simulink model "lab3s"  (R2025a)
settings: Solver=VariableStepAuto  StartTime=0.0  StopTime=15  MaxStep=5e-4  RelTol=1e-3
InitFcn:
  | clear;
  | 
  | % Plant Parameters
  | A = [0 1;-15 -7];
  | b0 = 3;
  | b = [0;3];
  | 
  | % Reference Model Parameters
  | c= 2;
  | tTa = 4.74;
  | tT= 0.7;
  | omega0 = tTa/tT;
  | 
  | am0 = omega0^2;
  | am1 = c * omega0;
  | Am = [0 1;-am0 -am1];
  | bm0 = am0;
  | bm = [0;bm0];
  | 
  | C = eye(2);
  | Q = eye(2);
  | 
  | % Controller Parameters
  | gamma =1;
  | P = lyap(Am',Q);
  | 
  | 
  | theta1 = (-am1 + A(2,1))/b0;
  | theta2 = (-am0 + A(2,2))/b0;
  | theta = [theta1;theta2];
settings Model: SimulationMode=accelerator  Creator=zuimio  LastModifiedBy=zuimio

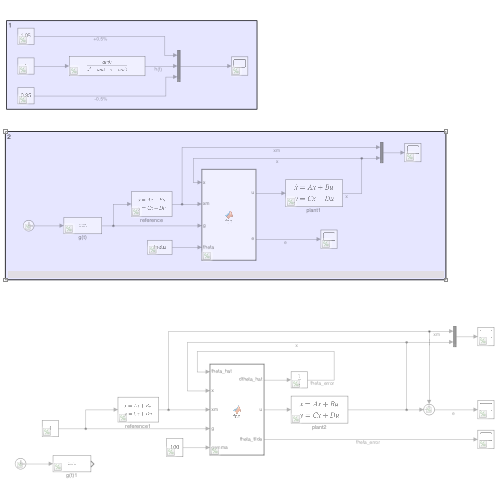
[thumbnail: Simulink's stored preview of the top-level diagram]
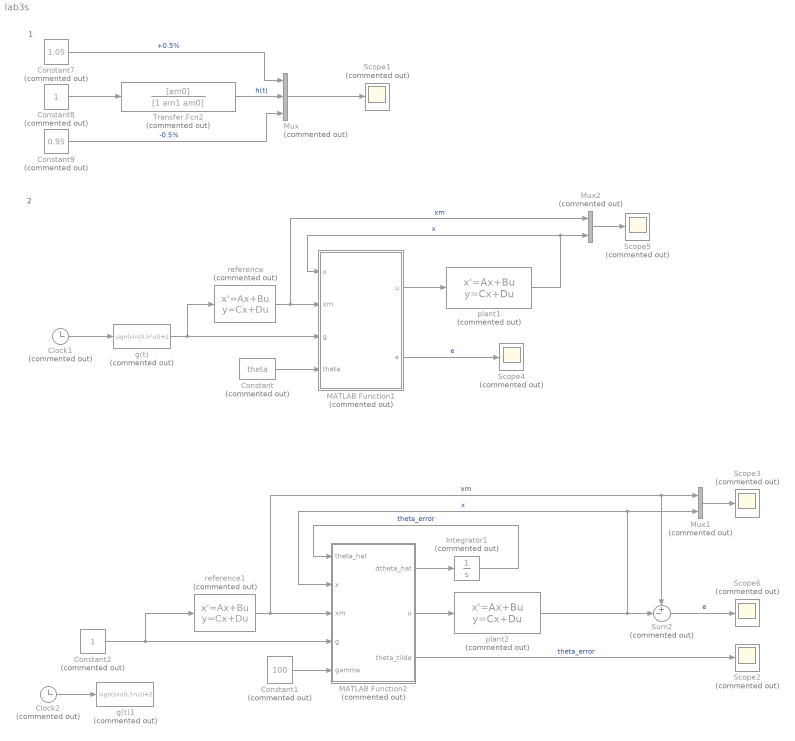
== system lab3s ==
  note: 2
  note: 1
  Clock1 : Clock  Commented=on
  Clock2 : Clock  Commented=on
  Constant : Constant  Commented=on  Value=theta
  Constant1 : Constant  Commented=on  Value=100
  Constant2 : Constant  Commented=on
  Constant7 : Constant  Commented=on  Value=1.05
  Constant8 : Constant  Commented=on
  Constant9 : Constant  Commented=on  Value=0.95
  Integrator1 : Integrator  Commented=on
  MATLAB Function1 : MATLAB Function  Commented=on  TreatAsAtomicUnit=on
  MATLAB Function2 : MATLAB Function  Commented=on  TreatAsAtomicUnit=on
  Mux : Mux  Commented=on  Inputs=3
  Mux1 : Mux  Commented=on  Inputs=2
  Mux2 : Mux  Commented=on  Inputs=2
  Scope{1..6} (6 alike) : Scope  Commented=on
      Scope1 settings: ActiveDisplayYMinimum=-0.13124999999999998  ActiveDisplayYMaximum=1.1812500000000001
      Scope2 settings: ActiveDisplayYMinimum=-19.8368626958697  ActiveDisplayYMaximum=2.3576146029633147
      Scope3 settings: ActiveDisplayYMinimum=-0.49074052302079013  ActiveDisplayYMaximum=3.7083192632435011  DataLoggingVariableName=ScopeData2
      Scope4 settings: ActiveDisplayYMinimum=-5.0922007223801344  ActiveDisplayYMaximum=7.0320573519139637  DataLoggingVariableName=ScopeData3
      Scope5 settings: ActiveDisplayYMinimum=-6.5390567265536914  ActiveDisplayYMaximum=9.0301156089836763  DataLoggingVariableName=ScopeData4
      Scope6 settings: ActiveDisplayYMinimum=-3.05730127485001  ActiveDisplayYMaximum=0.41335683185543448  DataLoggingVariableName=ScopeData5
  Sum2 : Sum  Commented=on  Inputs=+-|
  Transfer Fcn2 : TransferFcn  Commented=on  Numerator=[am0]  Denominator=[1 am1 am0]
  g(t) : MATLABFcn  Commented=on  MATLABFcn=sign(sin(0.5*u))+2
  g(t)1 : MATLABFcn  Commented=on  MATLABFcn=sign(sin(0.5*u))+2
  plant1 : StateSpace  Commented=on  A=A+[[0 0];[5 5]]  B=b  C=eye(2)  D=[0;0]  InitialCondition=[0;0]
  plant2 : StateSpace  Commented=on  A=A  B=b  C=eye(2)  D=[0;0]  InitialCondition=[0;0]
  reference : StateSpace  Commented=on  A=Am  B=bm  C=C  D=[0;0]  InitialCondition=[0;0]
  reference1 : StateSpace  Commented=on  A=Am  B=bm  C=C  D=[0;0]  InitialCondition=[0;0]
  wires:
  Transfer Fcn2/1 -> Mux/2  "h(t)"
  Mux/1 -> Scope1/1
  Constant9/1 -> Mux/3  "-0.5%"
  Constant8/1 -> Transfer Fcn2/1
  Constant7/1 -> Mux/1  "+0.5%"
  g(t)/1 -> reference/1, MATLAB Function1/3(g)
  reference/1 -> Mux2/1, MATLAB Function1/2(xm)  "xm"
  Clock1/1 -> g(t)/1
  Mux2/1 -> Scope5/1
  MATLAB Function1/1(u) -> plant1/1
  Constant1/1 -> MATLAB Function2/5(gamma)
  Mux1/1 -> Scope3/1
  plant2/1 -> Sum2/2, Mux1/2, MATLAB Function2/2(x)  "x"
  Clock2/1 -> g(t)1/1
  MATLAB Function2/1(dtheta_hat) -> Integrator1/1
  reference1/1 -> Mux1/1, Sum2/1, MATLAB Function2/3(xm)  "xm"
  Integrator1/1 -> MATLAB Function2/1(theta_hat)  "theta_error"
  Sum2/1 -> Scope6/1  "e"
  Constant/1 -> MATLAB Function1/4(theta)
  MATLAB Function1/2(e) -> Scope4/1  "e"
  MATLAB Function2/2(u) -> plant2/1
  plant1/1 -> Mux2/2, MATLAB Function1/1(x)  "x"
  MATLAB Function2/3(theta_tilde) -> Scope2/1  "theta_error"
  Constant2/1 -> reference1/1, MATLAB Function2/4(g)

== matlab function lab3s/MATLAB Function2 ==
  data: theta_hat input; dtheta_hat output; x input; xm input; g input; P parameter; b0 parameter; u output; am0 parameter; gamma input; b parameter; theta_tilde output; theta parameter
function [dtheta_hat, u, theta_tilde]  = fcn(theta_hat, x, xm, g, P, b0, am0, gamma, b, theta)
e = xm-x;
dtheta_hat = gamma * x * b' * P * e;
u = theta_hat' * x +  (am0/b0)*g;

theta_tilde = theta - theta_hat;

== matlab function lab3s/MATLAB Function1 ==
  data: x input; xm input; g input; u output; e output; theta input; b0 parameter; am0 parameter
function [u, e]  = fcn(x, xm, g, theta, b0, am0)
e = xm-x;
u = theta' * x +  (am0/b0)*g;
